simulink model "kangaroo"  (R2021b)
settings: Solver=VariableStepAuto  StartTime=0.0  StopTime=100  RelTol=1e-3
libraries: simulink x1
settings Model: Creator=Khaled  LastModifiedBy=Khaled

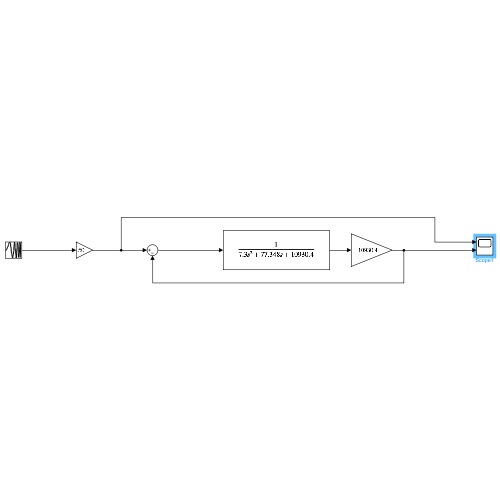
[thumbnail: Simulink's stored preview of the top-level diagram]
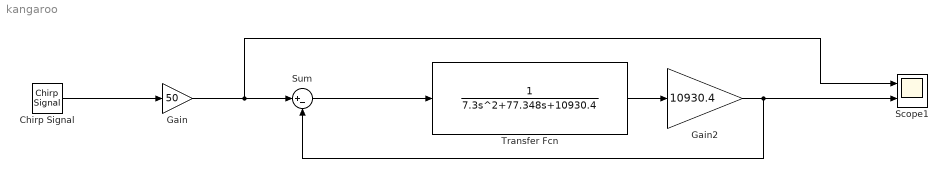
== system kangaroo ==
  Chirp Signal : simulink/Sources/Chirp Signal  f1=0.1  T=100  f2=1
  Gain : Gain  Gain=50
  Gain2 : Gain  Gain=10930.4
  Scope1 : Scope  NumInputPorts=2
  Sum : Sum  Inputs=|+-
  Transfer Fcn : TransferFcn  Denominator=[7.3 77.348 10930.4]
  wires:
  Gain2/1 -> Sum/2, Scope1/2
  Transfer Fcn/1 -> Gain2/1
  Gain/1 -> Scope1/1, Sum/1
  Sum/1 -> Transfer Fcn/1
  Chirp Signal/1 -> Gain/1
